simulink model "PRACTICA_03_P1_00"  (R2022a)
settings: Solver=VariableStepAuto  StartTime=0.0  StopTime=10.0  RelTol=1e-3
undefined symbols (not defined in the file or in its folder): xc7z010iclg225
libraries: hdlBasic x889, vmcUtilities x1
(part 1 of 4)
settings Model: Creator=sebas  LastModifiedBy=sebas

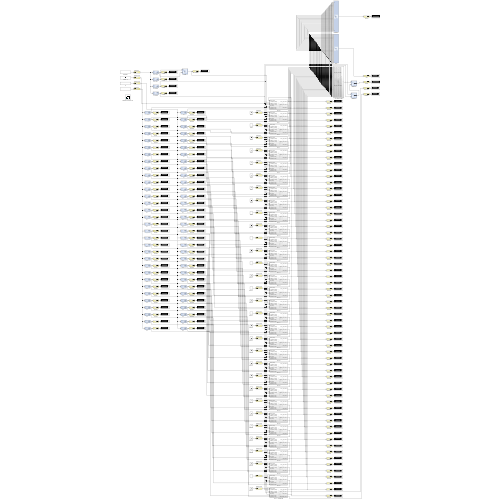
[thumbnail: Simulink's stored preview of the top-level diagram]
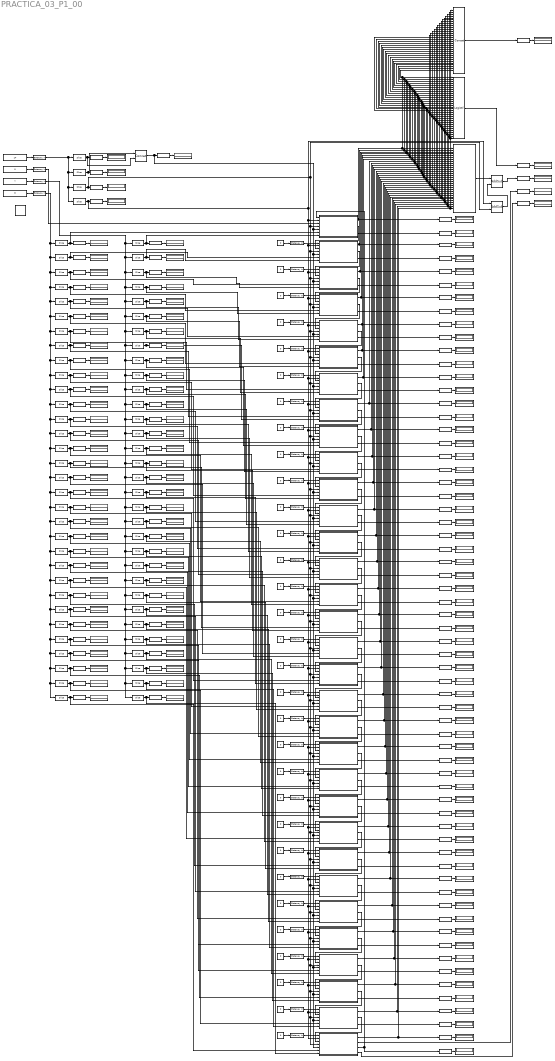
== system PRACTICA_03_P1_00 ==
  A : Constant  Value=8
  ALU_00 : Subsystem
  ALU_1 : Subsystem
  ALU_10 : Subsystem
  ALU_11 : Subsystem
  ALU_12 : Subsystem
  ALU_13 : Subsystem
  ALU_14 : Subsystem
  ALU_15 : Subsystem
  ALU_16 : Subsystem
  ALU_17 : Subsystem
  ALU_18 : Subsystem
  ALU_19 : Subsystem
  ALU_2 : Subsystem
  ALU_20 : Subsystem
  ALU_21 : Subsystem
  ALU_22 : Subsystem
  ALU_23 : Subsystem
  ALU_24 : Subsystem
  ALU_25 : Subsystem
  ALU_26 : Subsystem
  ALU_27 : Subsystem
  ALU_28 : Subsystem
  ALU_29 : Subsystem
  ALU_3 : Subsystem
  ALU_30 : Subsystem
  ALU_31_OVERFLOW : Subsystem
  ALU_4 : Subsystem
  ALU_5 : Subsystem
  ALU_6 : Subsystem
  ALU_7 : Subsystem
  ALU_8 : Subsystem
  ALU_9 : Subsystem
  ALU_OP_0 : hdlBasic/Slice  nbits=1  boolean_output=off  mode=Lower Bit Location + Width  bit1=-3  base1=MSB of Input  bit0=0  base0=LSB of Input  XmcBlockStatus=1  maskContainerNames=group1  block_type=slice  block_config=sysgen:Slice_config
  ALU_OP_1 : hdlBasic/Slice  nbits=1  boolean_output=off  mode=Lower Bit Location + Width  bit1=-2  base1=MSB of Input  bit0=1  base0=LSB of Input  XmcBlockStatus=1  maskContainerNames=group1  block_type=slice  block_config=sysgen:Slice_config
  ALU_OUT_32_BIT : Subsystem
  A_0 : hdlBasic/Slice  nbits=1  boolean_output=off  mode=Lower Bit Location + Width  bit1=-3  base1=MSB of Input  bit0=0  base0=LSB of Input  XmcBlockStatus=1  maskContainerNames=group1  block_type=slice  block_config=sysgen:Slice_config
  A_1 : hdlBasic/Slice  nbits=1  boolean_output=off  mode=Lower Bit Location + Width  bit1=-2  base1=MSB of Input  bit0=1  base0=LSB of Input  XmcBlockStatus=1  maskContainerNames=group1  block_type=slice  block_config=sysgen:Slice_config
  A_10 : hdlBasic/Slice  nbits=1  boolean_output=off  mode=Lower Bit Location + Width  bit1=-1  base1=MSB of Input  bit0=10  base0=LSB of Input  XmcBlockStatus=1  maskContainerNames=group1  block_type=slice  block_config=sysgen:Slice_config
  A_11 : hdlBasic/Slice  nbits=1  boolean_output=off  mode=Lower Bit Location + Width  bit1=0  base1=MSB of Input  bit0=11  base0=LSB of Input  XmcBlockStatus=1  maskContainerNames=group1  block_type=slice  block_config=sysgen:Slice_config
  A_12 : hdlBasic/Slice  nbits=1  boolean_output=off  mode=Lower Bit Location + Width  bit1=-3  base1=MSB of Input  bit0=12  base0=LSB of Input  XmcBlockStatus=1  maskContainerNames=group1  block_type=slice  block_config=sysgen:Slice_config
  A_13 : hdlBasic/Slice  nbits=1  boolean_output=off  mode=Lower Bit Location + Width  bit1=-2  base1=MSB of Input  bit0=13  base0=LSB of Input  XmcBlockStatus=1  maskContainerNames=group1  block_type=slice  block_config=sysgen:Slice_config
  A_14 : hdlBasic/Slice  nbits=1  boolean_output=off  mode=Lower Bit Location + Width  bit1=-1  base1=MSB of Input  bit0=14  base0=LSB of Input  XmcBlockStatus=1  maskContainerNames=group1  block_type=slice  block_config=sysgen:Slice_config
  A_15 : hdlBasic/Slice  nbits=1  boolean_output=off  mode=Lower Bit Location + Width  bit1=0  base1=MSB of Input  bit0=15  base0=LSB of Input  XmcBlockStatus=1  maskContainerNames=group1  block_type=slice  block_config=sysgen:Slice_config
  A_16 : hdlBasic/Slice  nbits=1  boolean_output=off  mode=Lower Bit Location + Width  bit1=-3  base1=MSB of Input  bit0=16  base0=LSB of Input  XmcBlockStatus=1  maskContainerNames=group1  block_type=slice  block_config=sysgen:Slice_config
  A_17 : hdlBasic/Slice  nbits=1  boolean_output=off  mode=Lower Bit Location + Width  bit1=-2  base1=MSB of Input  bit0=17  base0=LSB of Input  XmcBlockStatus=1  maskContainerNames=group1  block_type=slice  block_config=sysgen:Slice_config
  A_18 : hdlBasic/Slice  nbits=1  boolean_output=off  mode=Lower Bit Location + Width  bit1=-1  base1=MSB of Input  bit0=18  base0=LSB of Input  XmcBlockStatus=1  maskContainerNames=group1  block_type=slice  block_config=sysgen:Slice_config
  A_19 : hdlBasic/Slice  nbits=1  boolean_output=off  mode=Lower Bit Location + Width  bit1=0  base1=MSB of Input  bit0=19  base0=LSB of Input  XmcBlockStatus=1  maskContainerNames=group1  block_type=slice  block_config=sysgen:Slice_config
  A_2 : hdlBasic/Slice  nbits=1  boolean_output=off  mode=Lower Bit Location + Width  bit1=-1  base1=MSB of Input  bit0=2  base0=LSB of Input  XmcBlockStatus=1  maskContainerNames=group1  block_type=slice  block_config=sysgen:Slice_config
  A_20 : hdlBasic/Slice  nbits=1  boolean_output=off  mode=Lower Bit Location + Width  bit1=-3  base1=MSB of Input  bit0=20  base0=LSB of Input  XmcBlockStatus=1  maskContainerNames=group1  block_type=slice  block_config=sysgen:Slice_config
  A_21 : hdlBasic/Slice  nbits=1  boolean_output=off  mode=Lower Bit Location + Width  bit1=-2  base1=MSB of Input  bit0=21  base0=LSB of Input  XmcBlockStatus=1  maskContainerNames=group1  block_type=slice  block_config=sysgen:Slice_config
  A_22 : hdlBasic/Slice  nbits=1  boolean_output=off  mode=Lower Bit Location + Width  bit1=-1  base1=MSB of Input  bit0=22  base0=LSB of Input  XmcBlockStatus=1  maskContainerNames=group1  block_type=slice  block_config=sysgen:Slice_config
  A_23 : hdlBasic/Slice  nbits=1  boolean_output=off  mode=Lower Bit Location + Width  bit1=0  base1=MSB of Input  bit0=23  base0=LSB of Input  XmcBlockStatus=1  maskContainerNames=group1  block_type=slice  block_config=sysgen:Slice_config
  A_24 : hdlBasic/Slice  nbits=1  boolean_output=off  mode=Lower Bit Location + Width  bit1=-3  base1=MSB of Input  bit0=24  base0=LSB of Input  XmcBlockStatus=1  maskContainerNames=group1  block_type=slice  block_config=sysgen:Slice_config
  A_25 : hdlBasic/Slice  nbits=1  boolean_output=off  mode=Lower Bit Location + Width  bit1=-2  base1=MSB of Input  bit0=25  base0=LSB of Input  XmcBlockStatus=1  maskContainerNames=group1  block_type=slice  block_config=sysgen:Slice_config
  A_26 : hdlBasic/Slice  nbits=1  boolean_output=off  mode=Lower Bit Location + Width  bit1=-1  base1=MSB of Input  bit0=26  base0=LSB of Input  XmcBlockStatus=1  maskContainerNames=group1  block_type=slice  block_config=sysgen:Slice_config
  A_27 : hdlBasic/Slice  nbits=1  boolean_output=off  mode=Lower Bit Location + Width  bit1=0  base1=MSB of Input  bit0=27  base0=LSB of Input  XmcBlockStatus=1  maskContainerNames=group1  block_type=slice  block_config=sysgen:Slice_config
  A_28 : hdlBasic/Slice  nbits=1  boolean_output=off  mode=Lower Bit Location + Width  bit1=-3  base1=MSB of Input  bit0=28  base0=LSB of Input  XmcBlockStatus=1  maskContainerNames=group1  block_type=slice  block_config=sysgen:Slice_config
  A_29 : hdlBasic/Slice  nbits=1  boolean_output=off  mode=Lower Bit Location + Width  bit1=-2  base1=MSB of Input  bit0=29  base0=LSB of Input  XmcBlockStatus=1  maskContainerNames=group1  block_type=slice  block_config=sysgen:Slice_config
  A_3 : hdlBasic/Slice  nbits=1  boolean_output=off  mode=Lower Bit Location + Width  bit1=0  base1=MSB of Input  bit0=3  base0=LSB of Input  XmcBlockStatus=1  maskContainerNames=group1  block_type=slice  block_config=sysgen:Slice_config
  A_30 : hdlBasic/Slice  nbits=1  boolean_output=off  mode=Lower Bit Location + Width  bit1=-1  base1=MSB of Input  bit0=30  base0=LSB of Input  XmcBlockStatus=1  maskContainerNames=group1  block_type=slice  block_config=sysgen:Slice_config
  A_31 : hdlBasic/Slice  nbits=1  boolean_output=off  mode=Lower Bit Location + Width  bit1=0  base1=MSB of Input  bit0=31  base0=LSB of Input  XmcBlockStatus=1  maskContainerNames=group1  block_type=slice  block_config=sysgen:Slice_config
  A_4 : hdlBasic/Slice  nbits=1  boolean_output=off  mode=Lower Bit Location + Width  bit1=-3  base1=MSB of Input  bit0=4  base0=LSB of Input  XmcBlockStatus=1  maskContainerNames=group1  block_type=slice  block_config=sysgen:Slice_config
  A_5 : hdlBasic/Slice  nbits=1  boolean_output=off  mode=Lower Bit Location + Width  bit1=-2  base1=MSB of Input  bit0=5  base0=LSB of Input  XmcBlockStatus=1  maskContainerNames=group1  block_type=slice  block_config=sysgen:Slice_config
  A_6 : hdlBasic/Slice  nbits=1  boolean_output=off  mode=Lower Bit Location + Width  bit1=-1  base1=MSB of Input  bit0=6  base0=LSB of Input  XmcBlockStatus=1  maskContainerNames=group1  block_type=slice  block_config=sysgen:Slice_config
  A_7 : hdlBasic/Slice  nbits=1  boolean_output=off  mode=Lower Bit Location + Width  bit1=0  base1=MSB of Input  bit0=7  base0=LSB of Input  XmcBlockStatus=1  maskContainerNames=group1  block_type=slice  block_config=sysgen:Slice_config
  A_8 : hdlBasic/Slice  nbits=1  boolean_output=off  mode=Lower Bit Location + Width  bit1=-3  base1=MSB of Input  bit0=8  base0=LSB of Input  XmcBlockStatus=1  maskContainerNames=group1  block_type=slice  block_config=sysgen:Slice_config
  A_9 : hdlBasic/Slice  nbits=1  boolean_output=off  mode=Lower Bit Location + Width  bit1=-2  base1=MSB of Input  bit0=9  base0=LSB of Input  XmcBlockStatus=1  maskContainerNames=group1  block_type=slice  block_config=sysgen:Slice_config
  A_INVERT : hdlBasic/Slice  nbits=1  boolean_output=off  mode=Lower Bit Location + Width  bit1=0  base1=MSB of Input  bit0=3  base0=LSB of Input  XmcBlockStatus=1  maskContainerNames=group1  block_type=slice  block_config=sysgen:Slice_config
  AddSub1 : hdlBasic/AddSub  mode=Addition  use_carryin=off  use_carryout=off  en=off  latency=0  precision=User Defined  arith_type="Signed  (2's comp)"  n_bits=32  bin_pt=0  quantization=Truncate  overflow=Wrap  use_behavioral_HDL=off  hw_selection=Fabric  pipelined=off  XmcBlockStatus=1  maskContainerNames=tabcontainer1  block_type=addsub  block_config=sysgen:Addsub_config
  AddSub2 : hdlBasic/AddSub  mode=Addition  use_carryin=off  use_carryout=off  en=off  latency=0  precision=User Defined  arith_type="Signed  (2's comp)"  n_bits=32  bin_pt=0  quantization=Truncate  overflow=Wrap  use_behavioral_HDL=off  hw_selection=Fabric  pipelined=off  XmcBlockStatus=1  maskContainerNames=tabcontainer1  block_type=addsub  block_config=sysgen:Addsub_config
  B : Constant  Value=7
  B_0 : hdlBasic/Slice  nbits=1  boolean_output=off  mode=Lower Bit Location + Width  bit1=-3  base1=MSB of Input  bit0=0  base0=LSB of Input  XmcBlockStatus=1  maskContainerNames=group1  block_type=slice  block_config=sysgen:Slice_config
  B_1 : hdlBasic/Slice  nbits=1  boolean_output=off  mode=Lower Bit Location + Width  bit1=-2  base1=MSB of Input  bit0=1  base0=LSB of Input  XmcBlockStatus=1  maskContainerNames=group1  block_type=slice  block_config=sysgen:Slice_config
  B_10 : hdlBasic/Slice  nbits=1  boolean_output=off  mode=Lower Bit Location + Width  bit1=-1  base1=MSB of Input  bit0=10  base0=LSB of Input  XmcBlockStatus=1  maskContainerNames=group1  block_type=slice  block_config=sysgen:Slice_config
  B_11 : hdlBasic/Slice  nbits=1  boolean_output=off  mode=Lower Bit Location + Width  bit1=0  base1=MSB of Input  bit0=11  base0=LSB of Input  XmcBlockStatus=1  maskContainerNames=group1  block_type=slice  block_config=sysgen:Slice_config
  B_12 : hdlBasic/Slice  nbits=1  boolean_output=off  mode=Lower Bit Location + Width  bit1=-3  base1=MSB of Input  bit0=12  base0=LSB of Input  XmcBlockStatus=1  maskContainerNames=group1  block_type=slice  block_config=sysgen:Slice_config
  B_13 : hdlBasic/Slice  nbits=1  boolean_output=off  mode=Lower Bit Location + Width  bit1=-2  base1=MSB of Input  bit0=13  base0=LSB of Input  XmcBlockStatus=1  maskContainerNames=group1  block_type=slice  block_config=sysgen:Slice_config
  B_14 : hdlBasic/Slice  nbits=1  boolean_output=off  mode=Lower Bit Location + Width  bit1=-1  base1=MSB of Input  bit0=14  base0=LSB of Input  XmcBlockStatus=1  maskContainerNames=group1  block_type=slice  block_config=sysgen:Slice_config
  B_15 : hdlBasic/Slice  nbits=1  boolean_output=off  mode=Lower Bit Location + Width  bit1=0  base1=MSB of Input  bit0=15  base0=LSB of Input  XmcBlockStatus=1  maskContainerNames=group1  block_type=slice  block_config=sysgen:Slice_config
  B_16 : hdlBasic/Slice  nbits=1  boolean_output=off  mode=Lower Bit Location + Width  bit1=-3  base1=MSB of Input  bit0=16  base0=LSB of Input  XmcBlockStatus=1  maskContainerNames=group1  block_type=slice  block_config=sysgen:Slice_config
  B_17 : hdlBasic/Slice  nbits=1  boolean_output=off  mode=Lower Bit Location + Width  bit1=-2  base1=MSB of Input  bit0=17  base0=LSB of Input  XmcBlockStatus=1  maskContainerNames=group1  block_type=slice  block_config=sysgen:Slice_config
  B_18 : hdlBasic/Slice  nbits=1  boolean_output=off  mode=Lower Bit Location + Width  bit1=-1  base1=MSB of Input  bit0=18  base0=LSB of Input  XmcBlockStatus=1  maskContainerNames=group1  block_type=slice  block_config=sysgen:Slice_config
  B_19 : hdlBasic/Slice  nbits=1  boolean_output=off  mode=Lower Bit Location + Width  bit1=0  base1=MSB of Input  bit0=19  base0=LSB of Input  XmcBlockStatus=1  maskContainerNames=group1  block_type=slice  block_config=sysgen:Slice_config
  B_2 : hdlBasic/Slice  nbits=1  boolean_output=off  mode=Lower Bit Location + Width  bit1=-1  base1=MSB of Input  bit0=2  base0=LSB of Input  XmcBlockStatus=1  maskContainerNames=group1  block_type=slice  block_config=sysgen:Slice_config
  B_20 : hdlBasic/Slice  nbits=1  boolean_output=off  mode=Lower Bit Location + Width  bit1=-3  base1=MSB of Input  bit0=20  base0=LSB of Input  XmcBlockStatus=1  maskContainerNames=group1  block_type=slice  block_config=sysgen:Slice_config
  B_21 : hdlBasic/Slice  nbits=1  boolean_output=off  mode=Lower Bit Location + Width  bit1=-2  base1=MSB of Input  bit0=21  base0=LSB of Input  XmcBlockStatus=1  maskContainerNames=group1  block_type=slice  block_config=sysgen:Slice_config
  B_22 : hdlBasic/Slice  nbits=1  boolean_output=off  mode=Lower Bit Location + Width  bit1=-1  base1=MSB of Input  bit0=22  base0=LSB of Input  XmcBlockStatus=1  maskContainerNames=group1  block_type=slice  block_config=sysgen:Slice_config
  B_23 : hdlBasic/Slice  nbits=1  boolean_output=off  mode=Lower Bit Location + Width  bit1=0  base1=MSB of Input  bit0=23  base0=LSB of Input  XmcBlockStatus=1  maskContainerNames=group1  block_type=slice  block_config=sysgen:Slice_config
  B_24 : hdlBasic/Slice  nbits=1  boolean_output=off  mode=Lower Bit Location + Width  bit1=-3  base1=MSB of Input  bit0=24  base0=LSB of Input  XmcBlockStatus=1  maskContainerNames=group1  block_type=slice  block_config=sysgen:Slice_config
  B_25 : hdlBasic/Slice  nbits=1  boolean_output=off  mode=Lower Bit Location + Width  bit1=-2  base1=MSB of Input  bit0=25  base0=LSB of Input  XmcBlockStatus=1  maskContainerNames=group1  block_type=slice  block_config=sysgen:Slice_config
  B_26 : hdlBasic/Slice  nbits=1  boolean_output=off  mode=Lower Bit Location + Width  bit1=-1  base1=MSB of Input  bit0=26  base0=LSB of Input  XmcBlockStatus=1  maskContainerNames=group1  block_type=slice  block_config=sysgen:Slice_config
  B_27 : hdlBasic/Slice  nbits=1  boolean_output=off  mode=Lower Bit Location + Width  bit1=0  base1=MSB of Input  bit0=27  base0=LSB of Input  XmcBlockStatus=1  maskContainerNames=group1  block_type=slice  block_config=sysgen:Slice_config
  B_28 : hdlBasic/Slice  nbits=1  boolean_output=off  mode=Lower Bit Location + Width  bit1=-3  base1=MSB of Input  bit0=28  base0=LSB of Input  XmcBlockStatus=1  maskContainerNames=group1  block_type=slice  block_config=sysgen:Slice_config
  B_29 : hdlBasic/Slice  nbits=1  boolean_output=off  mode=Lower Bit Location + Width  bit1=-2  base1=MSB of Input  bit0=29  base0=LSB of Input  XmcBlockStatus=1  maskContainerNames=group1  block_type=slice  block_config=sysgen:Slice_config
  B_3 : hdlBasic/Slice  nbits=1  boolean_output=off  mode=Lower Bit Location + Width  bit1=0  base1=MSB of Input  bit0=3  base0=LSB of Input  XmcBlockStatus=1  maskContainerNames=group1  block_type=slice  block_config=sysgen:Slice_config
  B_30 : hdlBasic/Slice  nbits=1  boolean_output=off  mode=Lower Bit Location + Width  bit1=-1  base1=MSB of Input  bit0=30  base0=LSB of Input  XmcBlockStatus=1  maskContainerNames=group1  block_type=slice  block_config=sysgen:Slice_config
  B_31 : hdlBasic/Slice  nbits=1  boolean_output=off  mode=Lower Bit Location + Width  bit1=0  base1=MSB of Input  bit0=31  base0=LSB of Input  XmcBlockStatus=1  maskContainerNames=group1  block_type=slice  block_config=sysgen:Slice_config
  B_4 : hdlBasic/Slice  nbits=1  boolean_output=off  mode=Lower Bit Location + Width  bit1=-3  base1=MSB of Input  bit0=4  base0=LSB of Input  XmcBlockStatus=1  maskContainerNames=group1  block_type=slice  block_config=sysgen:Slice_config
  B_5 : hdlBasic/Slice  nbits=1  boolean_output=off  mode=Lower Bit Location + Width  bit1=-2  base1=MSB of Input  bit0=5  base0=LSB of Input  XmcBlockStatus=1  maskContainerNames=group1  block_type=slice  block_config=sysgen:Slice_config
  B_6 : hdlBasic/Slice  nbits=1  boolean_output=off  mode=Lower Bit Location + Width  bit1=-1  base1=MSB of Input  bit0=6  base0=LSB of Input  XmcBlockStatus=1  maskContainerNames=group1  block_type=slice  block_config=sysgen:Slice_config
  B_7 : hdlBasic/Slice  nbits=1  boolean_output=off  mode=Lower Bit Location + Width  bit1=0  base1=MSB of Input  bit0=7  base0=LSB of Input  XmcBlockStatus=1  maskContainerNames=group1  block_type=slice  block_config=sysgen:Slice_config
  B_8 : hdlBasic/Slice  nbits=1  boolean_output=off  mode=Lower Bit Location + Width  bit1=-3  base1=MSB of Input  bit0=8  base0=LSB of Input  XmcBlockStatus=1  maskContainerNames=group1  block_type=slice  block_config=sysgen:Slice_config
  B_9 : hdlBasic/Slice  nbits=1  boolean_output=off  mode=Lower Bit Location + Width  bit1=-2  base1=MSB of Input  bit0=9  base0=LSB of Input  XmcBlockStatus=1  maskContainerNames=group1  block_type=slice  block_config=sysgen:Slice_config
  B_INVERT : hdlBasic/Slice  nbits=1  boolean_output=off  mode=Lower Bit Location + Width  bit1=-1  base1=MSB of Input  bit0=2  base0=LSB of Input  XmcBlockStatus=1  maskContainerNames=group1  block_type=slice  block_config=sysgen:Slice_config
  CARRY_IN : Constant  Value=0
  CONTROL : Constant  Value=14
  Concat : hdlBasic/Concat  num_inputs=2  XmcBlockStatus=1  maskContainerNames=group1  block_type=concat  block_config=sysgen:Concat_config
  Concat1 : hdlBasic/Concat  num_inputs=32  XmcBlockStatus=1  maskContainerNames=group1  block_type=concat  block_config=sysgen:Concat_config
  Display{1..72,75,104..105,107..169} (138 alike) : Display
      Display3 settings: Format=decimal (Stored Integer)
      Display75 settings: Format=decimal (Stored Integer)
  Gateway In{1..7,11..35} (32 alike) : hdlBasic/Gateway In  gui_display_data_type=Fixed-point  arith_type=Unsigned  n_bits=1  bin_pt=0  preci_type=Single  exp_width=8  frac_width=24  rows=1  columns=1  quantization="Round  (unbiased: +/- Inf)"  overflow=Saturate  period=1  UseAsADC=off  ADCChannel='1'  interface=None  automatic_assignment=on  address_offset=hex2dec('00')  intf_name=''  intf_description=''  default_value=0  timing_constraint=None  locs_specified=off  LOCs={}  io_standard={}  inherit_from_input=off  hdl_port=on  XmcBlockStatus=1  maskContainerNames=group4  block_type=gatewayin  block_config=sysgen:gateway_in_config  block_width_w=590  block_height_w=620  block_width=640  block_height=850
  Gateway In10 : hdlBasic/Gateway In  gui_display_data_type=Fixed-point  arith_type=Signed (2's comp)  n_bits=32  bin_pt=0  preci_type=Single  exp_width=8  frac_width=24  rows=1  columns=1  quantization="Round  (unbiased: +/- Inf)"  overflow=Saturate  period=1  UseAsADC=off  ADCChannel='1'  interface=None  automatic_assignment=on  address_offset=hex2dec('00')  intf_name=''  intf_description=''  default_value=0  timing_constraint=None  locs_specified=off  LOCs={}  io_standard={}  inherit_from_input=off  hdl_port=on  XmcBlockStatus=1  maskContainerNames=group4  block_type=gatewayin  block_config=sysgen:gateway_in_config  block_width_w=590  block_height_w=620  block_width=640  block_height=850
  Gateway In8 : hdlBasic/Gateway In  gui_display_data_type=Fixed-point  arith_type=Unsigned  n_bits=4  bin_pt=0  preci_type=Single  exp_width=8  frac_width=24  rows=1  columns=1  quantization="Round  (unbiased: +/- Inf)"  overflow=Saturate  period=1  UseAsADC=off  ADCChannel='1'  interface=None  automatic_assignment=on  address_offset=hex2dec('00')  intf_name=''  intf_description=''  default_value=0  timing_constraint=None  locs_specified=off  LOCs={}  io_standard={}  inherit_from_input=off  hdl_port=on  XmcBlockStatus=1  maskContainerNames=group4  block_type=gatewayin  block_config=sysgen:gateway_in_config  block_width_w=590  block_height_w=620  block_width=640  block_height=850
  Gateway In9 : hdlBasic/Gateway In  gui_display_data_type=Fixed-point  arith_type=Unsigned  n_bits=32  bin_pt=0  preci_type=Single  exp_width=8  frac_width=24  rows=1  columns=1  quantization="Round  (unbiased: +/- Inf)"  overflow=Saturate  period=1  UseAsADC=off  ADCChannel='1'  interface=None  automatic_assignment=on  address_offset=hex2dec('00')  intf_name=''  intf_description=''  default_value=0  timing_constraint=None  locs_specified=off  LOCs={}  io_standard={}  inherit_from_input=off  hdl_port=on  XmcBlockStatus=1  maskContainerNames=group4  block_type=gatewayin  block_config=sysgen:gateway_in_config  block_width_w=590  block_height_w=620  block_width=640  block_height=850
  LESS_{1..31} (31 alike) : Constant  Value=0
  OP_2_BITS : hdlBasic/Gateway Out  inherit_from_input=off  hdl_port=on  rows=1  columns=1  UseAsDAC=off  DACChannel='1'  interface=None  automatic_assignment=on  address_offset=hex2dec('00')  intf_name=''  intf_description=''  timing_constraint=None  locs_specified=off  LOCs={}  io_standard={}  XmcBlockStatus=1  maskContainerNames=group4  block_type=gatewayout  block_config=sysgen:gateway_out_config  block_width_w=590  block_height_w=620  block_width=620  block_height=750
  Result{1..68,101,103..165} (132 alike) : hdlBasic/Gateway Out  inherit_from_input=off  hdl_port=on  rows=1  columns=1  UseAsDAC=off  DACChannel='1'  interface=None  automatic_assignment=on  address_offset=hex2dec('00')  intf_name=''  intf_description=''  timing_constraint=None  locs_specified=off  LOCs={}  io_standard={}  XmcBlockStatus=1  maskContainerNames=group4  block_type=gatewayout  block_config=sysgen:gateway_out_config  block_width_w=590  block_height_w=620  block_width=620  block_height=750
  Vitis Model Composer Hub : vmcUtilities/Vitis Model Composer Hub  Tag=genX  CodeGeneration=off  TargetDirectory=./code  ExportType=AI Engines  IpVendor=xilinx.com  IpLibrary=hls  IpVersion=1.0  IpHWLanguage=Verilog  AieCompilerOptions={}  AieSimulatorOptions={}  CreateTestbench=off  TestbenchStackSize=10  RunAieSim=off  AieSimTimeout=50000  RunAieSimProfiling=off  LaunchVitisAnalyzer=off  PlotOutput=off  RunX86Sim=off  X86SimTimeout=10  GenHwImage=off  PlatformType=Not Specified  HwSystemType=Baremetal  HwValidationTarget=hw  ProjDevice=xc7z010iclg225-1L  ProjDevicePart=xc7z010iclg225-1L  SamplePeriod=-1  ClockFrequency=200  DataPathParallelism=1  xilinxfamily=zynq  part=xc7z010i  speed=-1L  package=clg225  directory=./netlist  testbench=off  incr_netlist=off  synthesis_tool=Vivado  clock_wrapper=Clock Enables  dbl_ovrd=According to Block Masks  dcm_input_clock_period=10  sysclk_period=10  simulink_period=1  eval_field=0  LogFileName=''  NThreads=4
  _Carry_Out_ : hdlBasic/Gateway Out  inherit_from_input=off  hdl_port=on  rows=1  columns=1  UseAsDAC=off  DACChannel='1'  interface=None  automatic_assignment=on  address_offset=hex2dec('00')  intf_name=''  intf_description=''  timing_constraint=None  locs_specified=off  LOCs={}  io_standard={}  XmcBlockStatus=1  maskContainerNames=group4  block_type=gatewayout  block_config=sysgen:gateway_out_config  block_width_w=590  block_height_w=620  block_width=620  block_height=750
  _Overflow : hdlBasic/Gateway Out  inherit_from_input=off  hdl_port=on  rows=1  columns=1  UseAsDAC=off  DACChannel='1'  interface=None  automatic_assignment=on  address_offset=hex2dec('00')  intf_name=''  intf_description=''  timing_constraint=None  locs_specified=off  LOCs={}  io_standard={}  XmcBlockStatus=1  maskContainerNames=group4  block_type=gatewayout  block_config=sysgen:gateway_out_config  block_width_w=590  block_height_w=620  block_width=620  block_height=750
  _Result : hdlBasic/Gateway Out  inherit_from_input=off  hdl_port=on  rows=1  columns=1  UseAsDAC=off  DACChannel='1'  interface=None  automatic_assignment=on  address_offset=hex2dec('00')  intf_name=''  intf_description=''  timing_constraint=None  locs_specified=off  LOCs={}  io_standard={}  XmcBlockStatus=1  maskContainerNames=group4  block_type=gatewayout  block_config=sysgen:gateway_out_config  block_width_w=590  block_height_w=620  block_width=620  block_height=750
  _Result1 : hdlBasic/Gateway Out  inherit_from_input=off  hdl_port=on  rows=1  columns=1  UseAsDAC=off  DACChannel='1'  interface=None  automatic_assignment=on  address_offset=hex2dec('00')  intf_name=''  intf_description=''  timing_constraint=None  locs_specified=off  LOCs={}  io_standard={}  XmcBlockStatus=1  maskContainerNames=group4  block_type=gatewayout  block_config=sysgen:gateway_out_config  block_width_w=590  block_height_w=620  block_width=620  block_height=750
  _Zero : hdlBasic/Gateway Out  inherit_from_input=off  hdl_port=on  rows=1  columns=1  UseAsDAC=off  DACChannel='1'  interface=None  automatic_assignment=on  address_offset=hex2dec('00')  intf_name=''  intf_description=''  timing_constraint=None  locs_specified=off  LOCs={}  io_standard={}  XmcBlockStatus=1  maskContainerNames=group4  block_type=gatewayout  block_config=sysgen:gateway_out_config  block_width_w=590  block_height_w=620  block_width=620  block_height=750
  zero? : hdlBasic/Logical  logical_function=OR  inputs=32  en=off  latency=0  precision=Full  arith_type=Unsigned  n_bits=16  bin_pt=0  align_bp=on  overflow=[]  quantization=[]  XmcBlockStatus=1  maskContainerNames=tabcontainer1  block_type=logical  block_config=sysgen:Logical_config
  wires:
  Result2/1 -> Display5/1
  CONTROL/1 -> Gateway In8/1
  Gateway In8/1 -> A_INVERT/1, B_INVERT/1, ALU_OP_1/1, ALU_OP_0/1
  ALU_OP_0/1 -> Concat/2, Result2/1
  ALU_OP_1/1 -> Concat/1, Result1/1
  Result1/1 -> Display4/1
  B_INVERT/1 -> AddSub1/2, ALU_1/4(B_INVERT (1 BIT)), ALU_2/4(B_INVERT (1 BIT)), ALU_3/4(B_INVERT (1 BIT)), ALU_4/4(B_INVERT (1 BIT)), ALU_5/4(B_INVERT (1 BIT)), ALU_6/4(B_INVERT (1 BIT)), ALU_7/4(B_INVERT (1 BIT)), ALU_8/4(B_INVERT (1 BIT)), ALU_9/4(B_INVERT (1 BIT)), ALU_10/4(B_INVERT (1 BIT)), ALU_11/4(B_INVERT (1 BIT)), ALU_12/4(B_INVERT (1 BIT)), ALU_13/4(B_INVERT (1 BIT)), ALU_14/4(B_INVERT (1 BIT)), ALU_15/4(B_INVERT (1 BIT)), ALU_16/4(B_INVERT (1 BIT)), ALU_17/4(B_INVERT (1 BIT)), ALU_18/4(B_INVERT (1 BIT)), ALU_19/4(B_INVERT (1 BIT)), ALU_20/4(B_INVERT (1 BIT)), ALU_21/4(B_INVERT (1 BIT)), ALU_22/4(B_INVERT (1 BIT)), ALU_23/4(B_INVERT (1 BIT)), ALU_24/4(B_INVERT (1 BIT)), ALU_25/4(B_INVERT (1 BIT)), ALU_26/4(B_INVERT (1 BIT)), ALU_27/4(B_INVERT (1 BIT)), ALU_28/4(B_INVERT (1 BIT)), ALU_29/4(B_INVERT (1 BIT)), ALU_30/4(B_INVERT (1 BIT)), ALU_31_OVERFLOW/4(B_INVERT (1 BIT)), ALU_00/4(B_INVERT (1 BIT)), Result3/1
  Result3/1 -> Display6/1
  A_INVERT/1 -> AddSub1/1, ALU_1/2(A_INVERT (1 BIT)), ALU_2/2(A_INVERT (1 BIT)), ALU_3/2(A_INVERT (1 BIT)), ALU_4/2(A_INVERT (1 BIT)), ALU_5/2(A_INVERT (1 BIT)), ALU_6/2(A_INVERT (1 BIT)), ALU_7/2(A_INVERT (1 BIT)), ALU_8/2(A_INVERT (1 BIT)), ALU_9/2(A_INVERT (1 BIT)), ALU_10/2(A_INVERT (1 BIT)), ALU_11/2(A_INVERT (1 BIT)), ALU_12/2(A_INVERT (1 BIT)), ALU_13/2(A_INVERT (1 BIT)), ALU_14/2(A_INVERT (1 BIT)), ALU_15/2(A_INVERT (1 BIT)), ALU_16/2(A_INVERT (1 BIT)), ALU_17/2(A_INVERT (1 BIT)), ALU_18/2(A_INVERT (1 BIT)), ALU_19/2(A_INVERT (1 BIT)), ALU_20/2(A_INVERT (1 BIT)), ALU_21/2(A_INVERT (1 BIT)), ALU_22/2(A_INVERT (1 BIT)), ALU_23/2(A_INVERT (1 BIT)), ALU_24/2(A_INVERT (1 BIT)), ALU_25/2(A_INVERT (1 BIT)), ALU_26/2(A_INVERT (1 BIT)), ALU_27/2(A_INVERT (1 BIT)), ALU_28/2(A_INVERT (1 BIT)), ALU_29/2(A_INVERT (1 BIT)), ALU_30/2(A_INVERT (1 BIT)), ALU_31_OVERFLOW/2(A_INVERT (1 BIT)), ALU_00/2(A_INVERT (1 BIT)), Result4/1
  Result4/1 -> Display7/1
  A_0/1 -> ALU_00/6(A_INPUT (1 BIT)), Result6/1
  A_2/1 -> ALU_2/6(A_INPUT (1 BIT)), Result7/1
  Result5/1 -> Display8/1
  A_1/1 -> ALU_1/6(A_INPUT (1 BIT)), Result5/1
  A/1 -> Gateway In9/1
  Result6/1 -> Display9/1
  Result7/1 -> Display10/1
  Result8/1 -> Display11/1
  A_3/1 -> ALU_3/6(A_INPUT (1 BIT)), Result8/1
  Result11/1 -> Display12/1
  A_5/1 -> ALU_5/6(A_INPUT (1 BIT)), Result9/1
  Result9/1 -> Display14/1
  A_6/1 -> ALU_6/6(A_INPUT (1 BIT)), Result11/1
  Result10/1 -> Display15/1
  A_7/1 -> ALU_7/6(A_INPUT (1 BIT)), Result12/1
  Result12/1 -> Display13/1
  A_4/1 -> ALU_4/6(A_INPUT (1 BIT)), Result10/1
  Result15/1 -> Display16/1
  A_9/1 -> ALU_9/6(A_INPUT (1 BIT)), Result13/1
  Result13/1 -> Display18/1
  A_10/1 -> ALU_10/6(A_INPUT (1 BIT)), Result15/1
  Result14/1 -> Display19/1
  A_11/1 -> ALU_11/6(A_INPUT (1 BIT)), Result16/1
  Result16/1 -> Display17/1
  A_8/1 -> ALU_8/6(A_INPUT (1 BIT)), Result14/1
  Result19/1 -> Display20/1
  A_13/1 -> ALU_13/6(A_INPUT (1 BIT)), Result17/1
  Result17/1 -> Display22/1
  A_14/1 -> ALU_14/6(A_INPUT (1 BIT)), Result19/1
  Result18/1 -> Display23/1
  A_15/1 -> ALU_15/6(A_INPUT (1 BIT)), Result20/1
  Result20/1 -> Display21/1
  A_12/1 -> ALU_12/6(A_INPUT (1 BIT)), Result18/1
  A_17/1 -> ALU_17/6(A_INPUT (1 BIT)), Result21/1
  Result21/1 -> Display26/1
  Result22/1 -> Display27/1
  A_18/1 -> Result23/1, ALU_18/6(A_INPUT (1 BIT))
  A_19/1 -> ALU_19/6(A_INPUT (1 BIT)), Result24/1
  Result23/1 -> Display24/1
  Result24/1 -> Display25/1
  A_16/1 -> ALU_16/6(A_INPUT (1 BIT)), Result22/1
  A_21/1 -> ALU_21/6(A_INPUT (1 BIT)), Result25/1
  Result25/1 -> Display30/1
  Result26/1 -> Display31/1
  A_22/1 -> ALU_22/6(A_INPUT (1 BIT)), Result27/1
  A_23/1 -> ALU_23/6(A_INPUT (1 BIT)), Result28/1
  Result27/1 -> Display28/1
  Result28/1 -> Display29/1
  A_20/1 -> ALU_20/6(A_INPUT (1 BIT)), Result26/1
  A_25/1 -> ALU_25/6(A_INPUT (1 BIT)), Result29/1
  Result29/1 -> Display34/1
  Result30/1 -> Display35/1
  A_26/1 -> ALU_26/6(A_INPUT (1 BIT)), Result31/1
  A_27/1 -> ALU_27/6(A_INPUT (1 BIT)), Result32/1
  Result31/1 -> Display32/1
  Result32/1 -> Display33/1
  A_24/1 -> ALU_24/6(A_INPUT (1 BIT)), Result30/1
  A_29/1 -> ALU_29/6(A_INPUT (1 BIT)), Result33/1
  Result33/1 -> Display38/1
  Result34/1 -> Display39/1
  A_30/1 -> ALU_30/6(A_INPUT (1 BIT)), Result35/1
  A_31/1 -> ALU_31_OVERFLOW/6(A_INPUT (1 BIT)), Result36/1
  Result35/1 -> Display36/1
  Result36/1 -> Display37/1
  A_28/1 -> ALU_28/6(A_INPUT (1 BIT)), Result34/1
  Result39/1 -> Display43/1
  B_6/1 -> ALU_6/7(B_INPUT (1 BIT)), Result38/1
  B_5/1 -> ALU_5/7(B_INPUT (1 BIT)), Result68/1
  B_7/1 -> ALU_7/7(B_INPUT (1 BIT)), Result39/1
  Result37/1 -> Display45/1
  Result38/1 -> Display42/1
  B_20/1 -> ALU_20/7(B_INPUT (1 BIT)), Result53/1
  B_4/1 -> ALU_4/7(B_INPUT (1 BIT)), Result37/1
  B_13/1 -> ALU_13/7(B_INPUT (1 BIT)), Result44/1
  Result44/1 -> Display52/1
  B_14/1 -> ALU_14/7(B_INPUT (1 BIT)), Result46/1
  Result47/1 -> Display51/1
  B_12/1 -> ALU_12/7(B_INPUT (1 BIT)), Result45/1
  Result46/1 -> Display50/1
  Result68/1 -> Display44/1
  Result62/1 -> Display66/1
  Result63/1 -> Display67/1
  Result60/1 -> Display68/1
  Result61/1 -> Display69/1
  B_28/1 -> ALU_28/7(B_INPUT (1 BIT)), Result61/1
  B_31/1 -> ALU_31_OVERFLOW/7(B_INPUT (1 BIT)), Result63/1
  B_30/1 -> ALU_30/7(B_INPUT (1 BIT)), Result62/1
  B_29/1 -> ALU_29/7(B_INPUT (1 BIT)), Result60/1
  Result66/1 -> Display40/1
  B_2/1 -> ALU_2/7(B_INPUT (1 BIT)), Result66/1
  Result65/1 -> Display71/1
  Result67/1 -> Display41/1
  B/1 -> Gateway In10/1
  Result50/1 -> Display54/1
  Result51/1 -> Display55/1
  Result48/1 -> Display56/1
  Result64/1 -> Display70/1
  Result45/1 -> Display53/1
  B_19/1 -> ALU_19/7(B_INPUT (1 BIT)), Result51/1
  B_15/1 -> ALU_15/7(B_INPUT (1 BIT)), Result47/1
  B_24/1 -> ALU_24/7(B_INPUT (1 BIT)), Result57/1
  Result58/1 -> Display62/1
  B_27/1 -> ALU_27/7(B_INPUT (1 BIT)), Result59/1
  Result56/1 -> Display64/1
  B_25/1 -> ALU_25/7(B_INPUT (1 BIT)), Result56/1
  Result49/1 -> Display57/1
  B_11/1 -> ALU_11/7(B_INPUT (1 BIT)), Result43/1
  B_8/1 -> ALU_8/7(B_INPUT (1 BIT)), Result41/1
  Result57/1 -> Display65/1
  B_3/1 -> ALU_3/7(B_INPUT (1 BIT)), Result67/1
  Result40/1 -> Display48/1
  Result42/1 -> Display46/1
  B_9/1 -> ALU_9/7(B_INPUT (1 BIT)), Result40/1
  B_1/1 -> ALU_1/7(B_INPUT (1 BIT)), Result64/1
  Result41/1 -> Display49/1
  B_0/1 -> ALU_00/7(B_INPUT (1 BIT)), Result65/1
  B_16/1 -> ALU_16/7(B_INPUT (1 BIT)), Result49/1
  Result59/1 -> Display63/1
  B_18/1 -> ALU_18/7(B_INPUT (1 BIT)), Result50/1
  Result55/1 -> Display59/1
  Result53/1 -> Display61/1
  Result54/1 -> Display58/1
  Result43/1 -> Display47/1
  B_22/1 -> ALU_22/7(B_INPUT (1 BIT)), Result54/1
  Result52/1 -> Display60/1
  B_21/1 -> ALU_21/7(B_INPUT (1 BIT)), Result52/1
  B_10/1 -> ALU_10/7(B_INPUT (1 BIT)), Result42/1
  B_23/1 -> ALU_23/7(B_INPUT (1 BIT)), Result55/1
  B_17/1 -> ALU_17/7(B_INPUT (1 BIT)), Result48/1
  B_26/1 -> ALU_26/7(B_INPUT (1 BIT)), Result58/1
  CARRY_IN/1 -> Gateway In12/1
  Gateway In12/1 -> ALU_00/3(CARRY_IN (1 BIT))
  OP_2_BITS/1 -> Display104/1
  Concat/1 -> ALU_1/5(OP (2 BIT)), ALU_2/5(OP (2 BIT)), ALU_3/5(OP (2 BIT)), ALU_4/5(OP (2 BIT)), ALU_5/5(OP (2 BIT)), ALU_6/5(OP (2 BIT)), ALU_7/5(OP (2 BIT)), ALU_8/5(OP (2 BIT)), ALU_9/5(OP (2 BIT)), ALU_10/5(OP (2 BIT)), ALU_11/5(OP (2 BIT)), ALU_12/5(OP (2 BIT)), ALU_13/5(OP (2 BIT)), ALU_14/5(OP (2 BIT)), ALU_15/5(OP (2 BIT)), ALU_16/5(OP (2 BIT)), ALU_17/5(OP (2 BIT)), ALU_18/5(OP (2 BIT)), ALU_19/5(OP (2 BIT)), ALU_20/5(OP (2 BIT)), ALU_21/5(OP (2 BIT)), ALU_22/5(OP (2 BIT)), ALU_23/5(OP (2 BIT)), ALU_24/5(OP (2 BIT)), ALU_25/5(OP (2 BIT)), ALU_26/5(OP (2 BIT)), ALU_27/5(OP (2 BIT)), ALU_28/5(OP (2 BIT)), ALU_29/5(OP (2 BIT)), ALU_30/5(OP (2 BIT)), ALU_31_OVERFLOW/5(OP (2 BIT)), ALU_00/5(OP (2 BIT)), OP_2_BITS/1
  Result101/1 -> Display105/1
  ALU_00/1(ALU_OUT (1 BIT)) -> Result101/1, zero?/1, Concat1/32, ALU_OUT_32_BIT/1(ALU_OUT_0 (1 BIT))
  ALU_00/2(CARRY_OUT (1 BIT)) -> ALU_1/3(CARRY_IN (1 BIT))
  Result103/1 -> Display107/1
  ALU_00/3(SET (1 BIT)) -> Result103/1
  ALU_1/2(CARRY_OUT (1 BIT)) -> ALU_2/3(CARRY_IN (1 BIT))
  Result104/1 -> Display108/1
  ALU_1/1(ALU_OUT (1 BIT)) -> Result104/1, zero?/2, Concat1/31, ALU_OUT_32_BIT/2(ALU_OUT_1 (1 BIT))
  ALU_1/3(SET (1 BIT)) -> Result106/1
  Result106/1 -> Display110/1
  ALU_2/3(SET (1 BIT)) -> Result107/1
  ALU_2/1(ALU_OUT (1 BIT)) -> Result105/1, zero?/3, Concat1/30, ALU_OUT_32_BIT/3(ALU_OUT_2 (1 BIT))
  Result105/1 -> Display109/1
  Result107/1 -> Display111/1
  ALU_3/2(CARRY_OUT (1 BIT)) -> ALU_4/3(CARRY_IN (1 BIT))
  ALU_3/3(SET (1 BIT)) -> Result110/1
  Result110/1 -> Display114/1
  Result109/1 -> Display113/1
  ALU_3/1(ALU_OUT (1 BIT)) -> Result108/1, zero?/4, Concat1/29, ALU_OUT_32_BIT/4(ALU_OUT_3 (1 BIT))
  ALU_4/3(SET (1 BIT)) -> Result111/1
  ALU_4/1(ALU_OUT (1 BIT)) -> Result109/1, zero?/5, Concat1/28, ALU_OUT_32_BIT/5(ALU_OUT_4 (1 BIT))
  Result111/1 -> Display115/1
  Result108/1 -> Display112/1
  ALU_2/2(CARRY_OUT (1 BIT)) -> ALU_3/3(CARRY_IN (1 BIT))
  ALU_5/2(CARRY_OUT (1 BIT)) -> ALU_6/3(CARRY_IN (1 BIT))
  ALU_5/3(SET (1 BIT)) -> Result114/1
  Result114/1 -> Display118/1
  Result113/1 -> Display117/1
  ALU_5/1(ALU_OUT (1 BIT)) -> Result112/1, zero?/6, Concat1/27, ALU_OUT_32_BIT/6(ALU_OUT_5 (1 BIT))
  ALU_6/3(SET (1 BIT)) -> Result115/1
  ALU_6/1(ALU_OUT (1 BIT)) -> Result113/1, zero?/7, Concat1/26, ALU_OUT_32_BIT/7(ALU_OUT_6 (1 BIT))
  Result115/1 -> Display119/1
  Result112/1 -> Display116/1
  ALU_4/2(CARRY_OUT (1 BIT)) -> ALU_5/3(CARRY_IN (1 BIT))
  ALU_7/2(CARRY_OUT (1 BIT)) -> ALU_8/3(CARRY_IN (1 BIT))
  ALU_7/3(SET (1 BIT)) -> Result118/1
  Result118/1 -> Display122/1
  Result117/1 -> Display121/1
  ALU_7/1(ALU_OUT (1 BIT)) -> zero?/8, Concat1/25, ALU_OUT_32_BIT/8(ALU_OUT_7 (1 BIT)), Result116/1
  ALU_8/3(SET (1 BIT)) -> Result119/1
  ALU_8/1(ALU_OUT (1 BIT)) -> Result117/1, zero?/9, Concat1/24, ALU_OUT_32_BIT/9(ALU_OUT_8 (1 BIT))
  Result119/1 -> Display123/1
  Result116/1 -> Display120/1
  ALU_6/2(CARRY_OUT (1 BIT)) -> ALU_7/3(CARRY_IN (1 BIT))
  ALU_9/2(CARRY_OUT (1 BIT)) -> ALU_10/3(CARRY_IN (1 BIT))
  ALU_9/3(SET (1 BIT)) -> Result122/1
  Result122/1 -> Display126/1
  Result121/1 -> Display125/1
  ALU_9/1(ALU_OUT (1 BIT)) -> zero?/10, Concat1/23, ALU_OUT_32_BIT/10(ALU_OUT_9 (1 BIT)), Result120/1
  ALU_10/3(SET (1 BIT)) -> Result123/1
  ALU_10/1(ALU_OUT (1 BIT)) -> Result121/1, zero?/11, Concat1/22, ALU_OUT_32_BIT/11(ALU_OUT_10 (1 BIT))
  Result123/1 -> Display127/1
  Result120/1 -> Display124/1
  ALU_8/2(CARRY_OUT (1 BIT)) -> ALU_9/3(CARRY_IN (1 BIT))
  ALU_11/2(CARRY_OUT (1 BIT)) -> ALU_12/3(CARRY_IN (1 BIT))
  ALU_11/3(SET (1 BIT)) -> Result126/1
  Result126/1 -> Display130/1
  Result125/1 -> Display129/1
  ALU_11/1(ALU_OUT (1 BIT)) -> zero?/12, Concat1/21, ALU_OUT_32_BIT/12(ALU_OUT_11 (1 BIT)), Result124/1
  ALU_12/3(SET (1 BIT)) -> Result127/1
  ALU_12/1(ALU_OUT (1 BIT)) -> Result125/1, zero?/13, Concat1/20, ALU_OUT_32_BIT/13(ALU_OUT_12 (1 BIT))
  Result127/1 -> Display131/1
  Result124/1 -> Display128/1
  ALU_10/2(CARRY_OUT (1 BIT)) -> ALU_11/3(CARRY_IN (1 BIT))
  ALU_13/2(CARRY_OUT (1 BIT)) -> ALU_14/3(CARRY_IN (1 BIT))
  ALU_13/3(SET (1 BIT)) -> Result130/1
  Result130/1 -> Display134/1
  Result129/1 -> Display133/1
  ALU_13/1(ALU_OUT (1 BIT)) -> zero?/14, Concat1/19, ALU_OUT_32_BIT/14(ALU_OUT_13 (1 BIT)), Result128/1
  ALU_14/3(SET (1 BIT)) -> Result131/1
  ALU_14/1(ALU_OUT (1 BIT)) -> Result129/1, zero?/15, Concat1/18, ALU_OUT_32_BIT/15(ALU_OUT_14 (1 BIT))
  Result131/1 -> Display135/1
  Result128/1 -> Display132/1
  ALU_12/2(CARRY_OUT (1 BIT)) -> ALU_13/3(CARRY_IN (1 BIT))
  ALU_15/2(CARRY_OUT (1 BIT)) -> ALU_16/3(CARRY_IN (1 BIT))
  ALU_15/3(SET (1 BIT)) -> Result134/1
  Result134/1 -> Display138/1
  Result133/1 -> Display137/1
  ALU_15/1(ALU_OUT (1 BIT)) -> zero?/16, Concat1/17, ALU_OUT_32_BIT/16(ALU_OUT_15 (1 BIT)), Result132/1
  ALU_16/3(SET (1 BIT)) -> Result135/1
  ALU_16/1(ALU_OUT (1 BIT)) -> Result133/1, zero?/17, Concat1/16, ALU_OUT_32_BIT/17(ALU_OUT_16 (1 BIT))
  Result135/1 -> Display139/1
  Result132/1 -> Display136/1
  ALU_14/2(CARRY_OUT (1 BIT)) -> ALU_15/3(CARRY_IN (1 BIT))
  ALU_17/2(CARRY_OUT (1 BIT)) -> ALU_18/3(CARRY_IN (1 BIT))
  ALU_17/3(SET (1 BIT)) -> Result138/1
  Result138/1 -> Display142/1
  Result137/1 -> Display141/1
  ALU_17/1(ALU_OUT (1 BIT)) -> Concat1/15, zero?/18, ALU_OUT_32_BIT/18(ALU_OUT_17 (1 BIT)), Result136/1
  ALU_18/3(SET (1 BIT)) -> Result139/1
  ALU_18/1(ALU_OUT (1 BIT)) -> Result137/1, Concat1/14, zero?/19, ALU_OUT_32_BIT/19(ALU_OUT_18 (1 BIT))
  Result139/1 -> Display143/1
  Result136/1 -> Display140/1
  ALU_16/2(CARRY_OUT (1 BIT)) -> ALU_17/3(CARRY_IN (1 BIT))
  ALU_19/2(CARRY_OUT (1 BIT)) -> ALU_20/3(CARRY_IN (1 BIT))
  ALU_19/3(SET (1 BIT)) -> Result142/1
  Result142/1 -> Display146/1
  Result141/1 -> Display145/1
  ALU_19/1(ALU_OUT (1 BIT)) -> Concat1/13, zero?/20, ALU_OUT_32_BIT/20(ALU_OUT_19 (1 BIT)), Result140/1
  ALU_20/3(SET (1 BIT)) -> Result143/1
  ALU_20/1(ALU_OUT (1 BIT)) -> Result141/1, Concat1/12, zero?/21, ALU_OUT_32_BIT/21(ALU_OUT_20 (1 BIT))
  Result143/1 -> Display147/1
  Result140/1 -> Display144/1
  ALU_18/2(CARRY_OUT (1 BIT)) -> ALU_19/3(CARRY_IN (1 BIT))
  ALU_21/2(CARRY_OUT (1 BIT)) -> ALU_22/3(CARRY_IN (1 BIT))
  ALU_21/3(SET (1 BIT)) -> Result146/1
  Result146/1 -> Display150/1
  Result145/1 -> Display149/1
  ALU_21/1(ALU_OUT (1 BIT)) -> zero?/22, Concat1/11, ALU_OUT_32_BIT/22(ALU_OUT_21 (1 BIT)), Result144/1
  ALU_22/3(SET (1 BIT)) -> Result147/1
  ALU_22/1(ALU_OUT (1 BIT)) -> Result145/1, zero?/23, Concat1/10, ALU_OUT_32_BIT/23(ALU_OUT_22 (1 BIT))
  Result147/1 -> Display151/1
  Result144/1 -> Display148/1
  ALU_20/2(CARRY_OUT (1 BIT)) -> ALU_21/3(CARRY_IN (1 BIT))
  ALU_23/2(CARRY_OUT (1 BIT)) -> ALU_24/3(CARRY_IN (1 BIT))
  ALU_23/3(SET (1 BIT)) -> Result150/1
  Result150/1 -> Display154/1
  Result149/1 -> Display153/1
  ALU_23/1(ALU_OUT (1 BIT)) -> Concat1/9, zero?/24, ALU_OUT_32_BIT/24(ALU_OUT_23 (1 BIT)), Result148/1
  ALU_24/3(SET (1 BIT)) -> Result151/1
  ALU_24/1(ALU_OUT (1 BIT)) -> Result149/1, Concat1/8, zero?/25, ALU_OUT_32_BIT/25(ALU_OUT_24 (1 BIT))
  Result151/1 -> Display155/1
  Result148/1 -> Display152/1
  ALU_22/2(CARRY_OUT (1 BIT)) -> ALU_23/3(CARRY_IN (1 BIT))
  ALU_25/2(CARRY_OUT (1 BIT)) -> ALU_26/3(CARRY_IN (1 BIT))
  ALU_25/3(SET (1 BIT)) -> Result154/1
  Result154/1 -> Display158/1
  Result153/1 -> Display157/1
  ALU_25/1(ALU_OUT (1 BIT)) -> Concat1/7, zero?/26, ALU_OUT_32_BIT/26(ALU_OUT_25 (1 BIT)), Result152/1
  ALU_26/3(SET (1 BIT)) -> Result155/1
  ALU_26/1(ALU_OUT (1 BIT)) -> Result153/1, Concat1/6, zero?/27, ALU_OUT_32_BIT/27(ALU_OUT_26 (1 BIT))
  Result155/1 -> Display159/1
  Result152/1 -> Display156/1
  ALU_24/2(CARRY_OUT (1 BIT)) -> ALU_25/3(CARRY_IN (1 BIT))
  ALU_27/2(CARRY_OUT (1 BIT)) -> ALU_28/3(CARRY_IN (1 BIT))
  ALU_27/3(SET (1 BIT)) -> Result158/1
  Result158/1 -> Display162/1
  Result157/1 -> Display161/1
  ALU_27/1(ALU_OUT (1 BIT)) -> Concat1/5, zero?/28, ALU_OUT_32_BIT/28(ALU_OUT_27 (1 BIT)), Result156/1
  ALU_28/3(SET (1 BIT)) -> Result159/1
  ALU_28/1(ALU_OUT (1 BIT)) -> Result157/1, Concat1/4, zero?/29, ALU_OUT_32_BIT/29(ALU_OUT_28 (1 BIT))
  Result159/1 -> Display163/1
  Result156/1 -> Display160/1
  ALU_26/2(CARRY_OUT (1 BIT)) -> ALU_27/3(CARRY_IN (1 BIT))
  ALU_29/2(CARRY_OUT (1 BIT)) -> ALU_30/3(CARRY_IN (1 BIT))
  ALU_29/3(SET (1 BIT)) -> Result162/1
  Result162/1 -> Display166/1
  Result161/1 -> Display165/1
  ALU_29/1(ALU_OUT (1 BIT)) -> Concat1/3, zero?/30, ALU_OUT_32_BIT/30(ALU_OUT_29 (1 BIT)), Result160/1
  ALU_30/3(SET (1 BIT)) -> Result163/1
  ALU_30/1(ALU_OUT (1 BIT)) -> Result161/1, Concat1/2, zero?/31, ALU_OUT_32_BIT/31(ALU_OUT_30 (1 BIT))
  Result163/1 -> Display167/1
  Result160/1 -> Display164/1
  ALU_28/2(CARRY_OUT (1 BIT)) -> ALU_29/3(CARRY_IN (1 BIT))
  ALU_31_OVERFLOW/1(ALU_OUT (1 BIT)) -> zero?/32, Concat1/1, ALU_OUT_32_BIT/32(ALU_OUT_31 (1 BIT)), Result164/1
  ALU_31_OVERFLOW/3(SET (1 BIT)) -> Result165/1, ALU_00/1(LESS (1 BIT))
  Result165/1 -> Display169/1
  Result164/1 -> Display168/1
  ALU_30/2(CARRY_OUT (1 BIT)) -> ALU_31_OVERFLOW/3(CARRY_IN (1 BIT))
  LESS_1/1 -> Gateway In1/1
  Gateway In1/1 -> ALU_1/1(LESS (1 BIT))
  LESS_2/1 -> Gateway In2/1
  Gateway In2/1 -> ALU_2/1(LESS (1 BIT))
  LESS_3/1 -> Gateway In3/1
  Gateway In3/1 -> ALU_3/1(LESS (1 BIT))
  LESS_4/1 -> Gateway In4/1
  Gateway In4/1 -> ALU_4/1(LESS (1 BIT))
  LESS_5/1 -> Gateway In5/1
  Gateway In5/1 -> ALU_5/1(LESS (1 BIT))
  LESS_6/1 -> Gateway In6/1
  Gateway In6/1 -> ALU_6/1(LESS (1 BIT))
  LESS_7/1 -> Gateway In7/1
  Gateway In7/1 -> ALU_7/1(LESS (1 BIT))
  LESS_8/1 -> Gateway In11/1
  Gateway In11/1 -> ALU_8/1(LESS (1 BIT))
  LESS_9/1 -> Gateway In13/1
  Gateway In13/1 -> ALU_9/1(LESS (1 BIT))
  LESS_10/1 -> Gateway In14/1
  Gateway In14/1 -> ALU_10/1(LESS (1 BIT))
  LESS_11/1 -> Gateway In15/1
  Gateway In15/1 -> ALU_11/1(LESS (1 BIT))
  LESS_12/1 -> Gateway In16/1
  Gateway In16/1 -> ALU_12/1(LESS (1 BIT))
  LESS_13/1 -> Gateway In17/1
  Gateway In17/1 -> ALU_13/1(LESS (1 BIT))
  LESS_14/1 -> Gateway In18/1
  Gateway In18/1 -> ALU_14/1(LESS (1 BIT))
  LESS_15/1 -> Gateway In19/1
  Gateway In19/1 -> ALU_15/1(LESS (1 BIT))
  LESS_16/1 -> Gateway In20/1
  Gateway In20/1 -> ALU_16/1(LESS (1 BIT))
  LESS_17/1 -> Gateway In21/1
  Gateway In21/1 -> ALU_17/1(LESS (1 BIT))
  LESS_18/1 -> Gateway In22/1
  Gateway In22/1 -> ALU_18/1(LESS (1 BIT))
  LESS_19/1 -> Gateway In23/1
  Gateway In23/1 -> ALU_19/1(LESS (1 BIT))
  LESS_20/1 -> Gateway In24/1
  Gateway In24/1 -> ALU_20/1(LESS (1 BIT))
  LESS_21/1 -> Gateway In25/1
  Gateway In25/1 -> ALU_21/1(LESS (1 BIT))
  LESS_22/1 -> Gateway In26/1
  Gateway In26/1 -> ALU_22/1(LESS (1 BIT))
  LESS_23/1 -> Gateway In27/1
  Gateway In27/1 -> ALU_23/1(LESS (1 BIT))
  LESS_24/1 -> Gateway In28/1
  Gateway In28/1 -> ALU_24/1(LESS (1 BIT))
  LESS_25/1 -> Gateway In29/1
  Gateway In29/1 -> ALU_25/1(LESS (1 BIT))
  LESS_26/1 -> Gateway In30/1
  Gateway In30/1 -> ALU_26/1(LESS (1 BIT))
  LESS_27/1 -> Gateway In31/1
  Gateway In31/1 -> ALU_27/1(LESS (1 BIT))
  LESS_28/1 -> Gateway In32/1
  Gateway In32/1 -> ALU_28/1(LESS (1 BIT))
  LESS_29/1 -> Gateway In33/1
  Gateway In33/1 -> ALU_29/1(LESS (1 BIT))
  LESS_30/1 -> Gateway In34/1
  Gateway In34/1 -> ALU_30/1(LESS (1 BIT))
  LESS_31/1 -> Gateway In35/1
  Gateway In35/1 -> ALU_31_OVERFLOW/1(LESS (1 BIT))
  _Carry_Out_/1 -> Display1/1
  _Zero/1 -> Display2/1
  _Result/1 -> Display3/1
  ALU_31_OVERFLOW/2(CARRY_OUT (1 BIT)) -> _Carry_Out_/1
  zero?/1 -> _Zero/1
  _Overflow/1 -> Display72/1
  ALU_31_OVERFLOW/4(OVERFLOW (1 BIT)) -> _Overflow/1
  Gateway In9/1 -> A_31/1, A_30/1, A_29/1, A_28/1, A_27/1, A_26/1, A_25/1, A_24/1, A_23/1, A_22/1, A_21/1, A_20/1, A_19/1, A_18/1, A_17/1, A_16/1, A_15/1, A_14/1, A_13/1, A_12/1, A_11/1, A_10/1, A_9/1, A_8/1, A_7/1, A_6/1, A_5/1, A_4/1, A_3/1, A_2/1, A_1/1, A_0/1
  Gateway In10/1 -> B_31/1, B_30/1, B_29/1, B_28/1, B_27/1, B_26/1, B_25/1, B_24/1, B_23/1, B_22/1, B_21/1, B_20/1, B_19/1, B_18/1, B_17/1, B_16/1, B_15/1, B_14/1, B_13/1, B_12/1, B_11/1, B_10/1, B_9/1, B_8/1, B_7/1, B_6/1, B_5/1, B_4/1, B_3/1, B_2/1, B_1/1, B_0/1
  _Result1/1 -> Display75/1
  Concat1/1 -> _Result1/1
  AddSub1/1 -> AddSub2/2
  ALU_OUT_32_BIT/1(Out1) -> AddSub2/1
  AddSub2/1 -> _Result/1

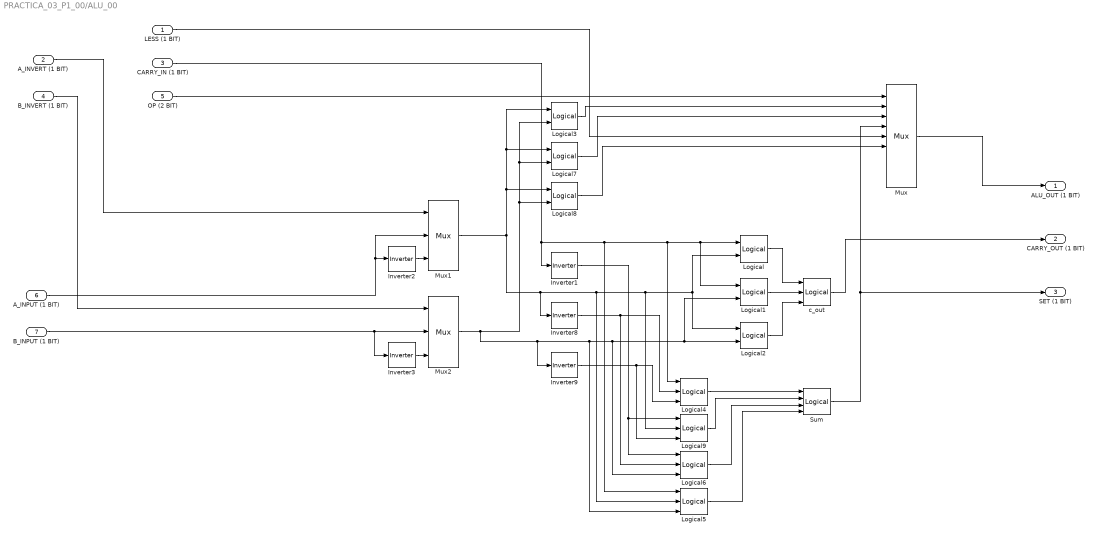
== system PRACTICA_03_P1_00/ALU_00 ==
  LESS (1 BIT) : Inport
  A_INVERT (1 BIT) : Inport  Port=2
  CARRY_IN (1 BIT) : Inport  Port=3
  B_INVERT (1 BIT) : Inport  Port=4
  OP (2 BIT) : Inport  Port=5
  A_INPUT (1 BIT) : Inport  Port=6
  B_INPUT (1 BIT) : Inport  Port=7
  Inverter{1..3,8..9} (5 alike) : hdlBasic/Inverter  en=off  latency=0  XmcBlockStatus=1  maskContainerNames=group2  block_type=inv  block_config=sysgen:Inverter_config
  Logical{,1..3} (4 alike) : hdlBasic/Logical  logical_function=AND  inputs=2  en=off  latency=0  precision=Full  arith_type=Unsigned  n_bits=16  bin_pt=0  align_bp=on  overflow=[]  quantization=[]  XmcBlockStatus=1  maskContainerNames=tabcontainer1  block_type=logical  block_config=sysgen:Logical_config
  Logical{4..6,9} (4 alike) : hdlBasic/Logical  logical_function=AND  inputs=3  en=off  latency=0  precision=Full  arith_type=Unsigned  n_bits=16  bin_pt=0  align_bp=on  overflow=[]  quantization=[]  XmcBlockStatus=1  maskContainerNames=tabcontainer1  block_type=logical  block_config=sysgen:Logical_config
  Logical7 : hdlBasic/Logical  logical_function=OR  inputs=2  en=off  latency=0  precision=Full  arith_type=Unsigned  n_bits=16  bin_pt=0  align_bp=on  overflow=[]  quantization=[]  XmcBlockStatus=1  maskContainerNames=tabcontainer1  block_type=logical  block_config=sysgen:Logical_config
  Logical8 : hdlBasic/Logical  logical_function=XOR  inputs=2  en=off  latency=0  precision=Full  arith_type=Unsigned  n_bits=16  bin_pt=0  align_bp=on  overflow=[]  quantization=[]  XmcBlockStatus=1  maskContainerNames=tabcontainer1  block_type=logical  block_config=sysgen:Logical_config
  Mux : hdlBasic/Mux  inputs=8  en=off  latency=0  precision=Full  arith_type=Unsigned  n_bits=16  bin_pt=14  quantization=Truncate  overflow=Wrap  XmcBlockStatus=1  maskContainerNames=tabcontainer1  block_type=mux  block_config=sysgen:Mux_config
  Mux1 : hdlBasic/Mux  inputs=2  en=off  latency=0  precision=Full  arith_type=Unsigned  n_bits=16  bin_pt=14  quantization=Truncate  overflow=Wrap  XmcBlockStatus=1  maskContainerNames=tabcontainer1  block_type=mux  block_config=sysgen:Mux_config
  Mux2 : hdlBasic/Mux  inputs=2  en=off  latency=0  precision=Full  arith_type=Unsigned  n_bits=16  bin_pt=14  quantization=Truncate  overflow=Wrap  XmcBlockStatus=1  maskContainerNames=tabcontainer1  block_type=mux  block_config=sysgen:Mux_config
  Sum : hdlBasic/Logical  logical_function=OR  inputs=4  en=off  latency=0  precision=Full  arith_type=Unsigned  n_bits=16  bin_pt=0  align_bp=on  overflow=[]  quantization=[]  XmcBlockStatus=1  maskContainerNames=tabcontainer1  block_type=logical  block_config=sysgen:Logical_config
  c_out : hdlBasic/Logical  logical_function=OR  inputs=3  en=off  latency=0  precision=Full  arith_type=Unsigned  n_bits=16  bin_pt=0  align_bp=on  overflow=[]  quantization=[]  XmcBlockStatus=1  maskContainerNames=tabcontainer1  block_type=logical  block_config=sysgen:Logical_config
  ALU_OUT (1 BIT) : Outport
  CARRY_OUT (1 BIT) : Outport  Port=2
  SET (1 BIT) : Outport  Port=3
  wires:
  Mux1/1 -> Logical8/1, Logical7/1, Logical3/1, Inverter8/1, Logical5/2, Logical/2, Logical2/1, Logical9/2
  Logical1/1 -> c_out/2
  Inverter8/1 -> Logical6/2, Logical4/2
  A_INPUT (1 BIT)/1 -> Mux1/2, Inverter2/1
  CARRY_IN (1 BIT)/1 -> Inverter1/1, Logical5/1, Logical4/1, Logical1/1, Logical/1
  Mux2/1 -> Logical5/3, Logical6/3, Logical1/2, Logical2/2, Inverter9/1, Logical8/2, Logical3/2, Logical7/2
  Inverter2/1 -> Mux1/3
  Inverter1/1 -> Logical6/1, Logical9/1
  Logical6/1 -> Sum/3
  B_INPUT (1 BIT)/1 -> Inverter3/1, Mux2/2
  Logical9/1 -> Sum/2
  Sum/1 -> SET (1 BIT)/1, Mux/4
  Logical4/1 -> Sum/1
  Inverter3/1 -> Mux2/3
  Logical7/1 -> Mux/3
  Logical/1 -> c_out/1
  Logical5/1 -> Sum/4
  Logical3/1 -> Mux/2
  Inverter9/1 -> Logical9/3, Logical4/3
  Mux/1 -> ALU_OUT (1 BIT)/1
  Logical2/1 -> c_out/3
  OP (2 BIT)/1 -> Mux/1
  A_INVERT (1 BIT)/1 -> Mux1/1
  B_INVERT (1 BIT)/1 -> Mux2/1
  c_out/1 -> CARRY_OUT (1 BIT)/1
  LESS (1 BIT)/1 -> Mux/5
  Logical8/1 -> Mux/6
